simulink model "L4_1"  (R2023a)
settings: Solver=VariableStepAuto  StartTime=0.0  StopTime=20  RelTol=1e-8
undefined symbols (not defined in the file): a0, a1, a2, k0, k1, T
settings Model: Creator=apere  LastModifiedBy=apere

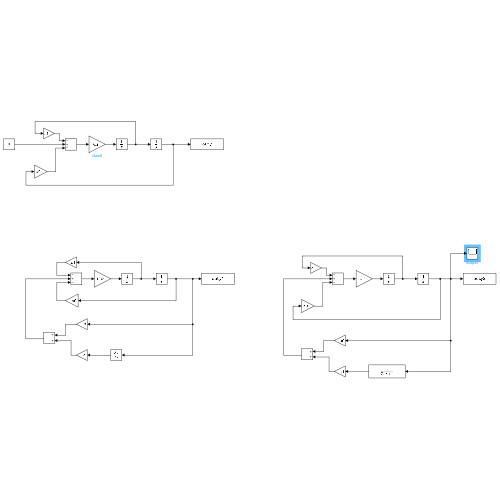
[thumbnail: Simulink's stored preview of the top-level diagram]
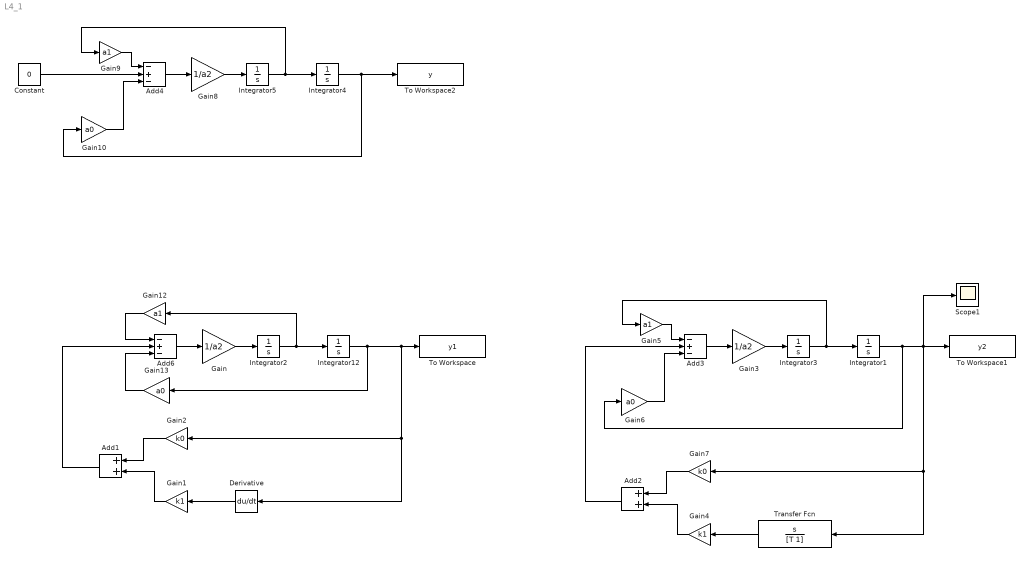
== system L4_1 ==
  Add1 : Sum
  Add2 : Sum
  Add3 : Sum  Inputs=-+-
  Add4 : Sum  Inputs=-+-
  Add6 : Sum  Inputs=-+-
  Constant : Constant  Value=0
  Derivative : Derivative
  Gain : Gain  Gain=1/a2
  Gain1 : Gain  Gain=k1
  Gain10 : Gain  Gain=a0
  Gain12 : Gain  Gain=a1
  Gain13 : Gain  Gain=a0
  Gain2 : Gain  Gain=k0
  Gain3 : Gain  Gain=1/a2
  Gain4 : Gain  Gain=k1
  Gain5 : Gain  Gain=a1
  Gain6 : Gain  Gain=a0
  Gain7 : Gain  Gain=k0
  Gain8 : Gain  Gain=1/a2
  Gain9 : Gain  Gain=a1
  Integrator{1..5,12} (6 alike) : Integrator  InitialCondition=1
  Scope1 : Scope
  To Workspace : ToWorkspace  VariableName=y1  SaveFormat=Timeseries  SampleTime=-1
  To Workspace1 : ToWorkspace  VariableName=y2  SaveFormat=Timeseries  SampleTime=-1
  To Workspace2 : ToWorkspace  VariableName=y  SaveFormat=Timeseries  SampleTime=-1
  Transfer Fcn : TransferFcn  Numerator=[1 0]  Denominator=[T 1]
  wires:
  Integrator12/1 -> To Workspace/1, Derivative/1, Gain2/1, Gain13/1
  Integrator2/1 -> Integrator12/1, Gain12/1
  Add1/1 -> Add6/2
  Gain13/1 -> Add6/3
  Gain12/1 -> Add6/1
  Derivative/1 -> Gain1/1
  Gain2/1 -> Add1/1
  Gain1/1 -> Add1/2
  Add6/1 -> Gain/1
  Gain/1 -> Integrator2/1
  Integrator1/1 -> Scope1/1, To Workspace1/1, Gain7/1, Transfer Fcn/1, Gain6/1
  Gain5/1 -> Add3/1
  Gain6/1 -> Add3/3
  Add3/1 -> Gain3/1
  Gain3/1 -> Integrator3/1
  Integrator3/1 -> Integrator1/1, Gain5/1
  Gain7/1 -> Add2/1
  Gain4/1 -> Add2/2
  Add2/1 -> Add3/2
  Transfer Fcn/1 -> Gain4/1
  Gain8/1 -> Integrator5/1
  Add4/1 -> Gain8/1
  Gain10/1 -> Add4/3
  Gain9/1 -> Add4/1
  Constant/1 -> Add4/2
  Integrator5/1 -> Integrator4/1, Gain9/1
  Integrator4/1 -> To Workspace2/1, Gain10/1
